simulink model "nonsim"  (Simulink 7.9)
settings: Solver=ode45  StartTime=0.0  StopTime=150.0  RelTol=1e-3
values from neighbouring files (symbols this model uses):
  a = [A, 0*A ... (first row only)    [fig10_21.m]    (also in fig10_22.m; fig10_23.m; fig10_24.m; fig10_38.m = [Apw, 0*Apw)
  N = reshape(xx(n*nm+1:end),p,nm)    [Modelfollowingdesign.m]    (also in f_tos.m = 1; fig10_18.m = S\r; fig10_19.m = S\r; fig10_20.m = S\r)
  r = rlocus(Aol,Bol,Col,Dol,k5)    [fig10_15.m]    (also in fig10_18.m = [0*B;1]; fig10_19.m = [0*B;1]; fig10_20.m = [0*B;1]; fig10_21.m = [0*B;1])
undefined symbols (not defined in the file or in its folder): den, df, nf, num
settings Model: Creator=abbas  LastModifiedBy=abbas  ExtModeTrigMode=oneshot  ExtModeArmWhenConnect=off
settings DataIOCC: LimitDataPoints=off
settings OptimizationCC: BlockReduction=off  BooleanDataType=off  InitFltsAndDblsToZero=on
settings DebuggingCC: SaveWithParameterizedLinksMsg=none  SignalResolutionControl=TryResolveAllWithWarning  SolverPrmCheckMsg=none  MultiTaskDSMMsg=warning  MultiTaskCondExecSysMsg=none  FcnCallInpInsideContextMsg=Use local settings  StrictBusMsg=None
settings HardwareCC: TargetUnknown=on
settings RTWCC: IncludeERTFirstTime=on
settings GRTTargetCC: ModelReferenceCompliant=off  CompOptLevelCompliant=off  CombineOutputUpdateFcns=off  MatFileLogging=off  GRTInterface=on

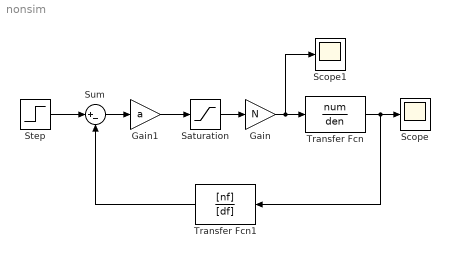
== system nonsim ==
  Gain : Gain  Gain=N  SaturateOnIntegerOverflow=on  OutDataTypeStr=Inherit: Same as input  ParamDataTypeStr=Inherit: Same as input
  Gain1 : Gain  Gain=a  SaturateOnIntegerOverflow=on  OutDataTypeStr=Inherit: Same as input  ParamDataTypeStr=Inherit: Same as input
  Saturation : Saturate  UpperLimit=1  LowerLimit=-1
  Scope : Scope
      settings: SaveName=yn
  Scope1 : Scope
      settings: SaveName=yn1
  Step : Step  Time=.1  After=r  SampleTime=0.01
  Sum : Sum  Inputs=|+-  SaturateOnIntegerOverflow=on  InputSameDT=on  OutDataTypeStr=Inherit: Same as first input
  Transfer Fcn : TransferFcn  Numerator=num  Denominator=den
  Transfer Fcn1 : TransferFcn  Numerator=[nf]  Denominator=[df]
  wires:
  Step/1 -> Sum/1
  Gain1/1 -> Saturation/1
  Sum/1 -> Gain1/1
  Saturation/1 -> Gain/1
  Gain/1 -> Transfer Fcn/1, Scope1/1
  Transfer Fcn/1 -> Scope/1, Transfer Fcn1/1
  Transfer Fcn1/1 -> Sum/2
